simulink model "threebitsynupdowncounter"  (R2024a)
settings: Solver=VariableStepAuto  StartTime=0.0  StopTime=10.0  RelTol=1e-3
libraries: simulink_extras x4
settings Model: Creator=prath  LastModifiedBy=prath

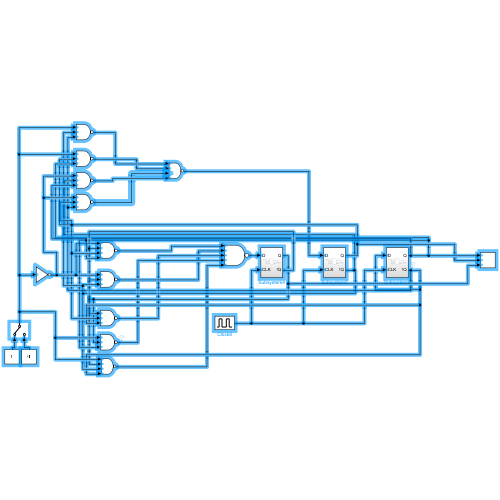
[thumbnail: Simulink's stored preview of the top-level diagram]
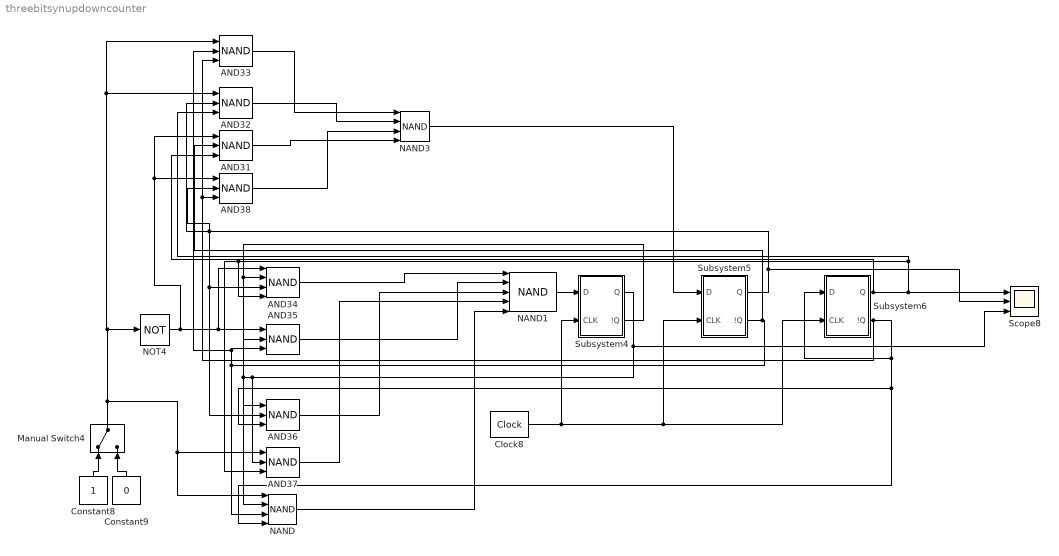
== system threebitsynupdowncounter ==
  AND{31..33,35..38} (7 alike) : Logic  Operator=NAND  Inputs=3  IconShape=distinctive  AllPortsSameDT=off  OutDataTypeStr=boolean
  AND34 : Logic  Operator=NAND  Inputs=4  IconShape=distinctive  AllPortsSameDT=off  OutDataTypeStr=boolean
  Clock8 : simulink_extras/Flip Flops/Clock  period=0.5
  Constant8 : Constant  OutDataTypeStr=boolean
  Constant9 : Constant  Value=0  OutDataTypeStr=boolean
  Manual Switch4 : ManualSwitch
  NAND : Logic  Operator=NAND  Inputs=4  IconShape=distinctive  AllPortsSameDT=off  OutDataTypeStr=boolean
  NAND1 : Logic  Operator=NAND  Inputs=5  IconShape=distinctive  AllPortsSameDT=off  OutDataTypeStr=boolean
  NAND3 : Logic  Operator=NAND  Inputs=4  IconShape=distinctive  AllPortsSameDT=off  OutDataTypeStr=boolean
  NOT4 : Logic  Operator=NOT  IconShape=distinctive  AllPortsSameDT=off  OutDataTypeStr=boolean
  Scope8 : Scope  NumInputPorts=3
  Subsystem4 : Subsystem
  Subsystem5 : Subsystem
  Subsystem6 : Subsystem
  wires:
  NAND/1 -> NAND1/5
  Clock8/1 -> Subsystem6/2(CLK), Subsystem5/2(CLK), Subsystem4/2(CLK)
  Subsystem5/2(!Q) -> AND31/2, AND35/3, AND33/2, NAND/3
  NOT4/1 -> AND38/1, AND31/1, AND35/1, AND34/1
  Subsystem5/1(Q) -> Scope8/2, AND32/2, AND36/2, AND34/3, AND38/2
  AND33/1 -> NAND3/1
  NAND3/1 -> Subsystem5/1(D)
  Subsystem6/2(!Q) -> AND38/3, AND33/3, AND36/3, NAND/4, Subsystem6/1(D)
  Manual Switch4/1 -> AND37/1, NAND/1, NOT4/1, AND32/1, AND33/1
  NAND1/1 -> Subsystem4/1(D)
  Subsystem6/1(Q) -> AND31/3, AND34/4, AND37/3, AND32/3, Scope8/1
  AND31/1 -> NAND3/4
  AND35/1 -> NAND1/2
  Constant9/1 -> Manual Switch4/2
  AND34/1 -> NAND1/1
  AND36/1 -> NAND1/3
  Subsystem4/1(Q) -> Scope8/3, AND37/2, AND36/1, AND35/2
  AND37/1 -> NAND1/4
  Subsystem4/2(!Q) -> NAND/2, AND34/2
  Constant8/1 -> Manual Switch4/1
  AND32/1 -> NAND3/2
  AND38/1 -> NAND3/3

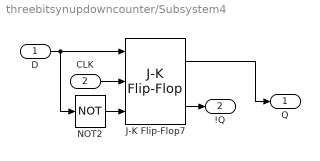
== system threebitsynupdowncounter/Subsystem4 ==
  D : Inport
  CLK : Inport  Port=2
  J-K Flip-Flop7 : simulink_extras/Flip Flops/J-K Flip-Flop  initial_condition=0
  NOT2 : Logic  Operator=NOT  IconShape=distinctive  AllPortsSameDT=off  OutDataTypeStr=boolean
  Q : Outport
  !Q : Outport  Port=2
  wires:
  NOT2/1 -> J-K Flip-Flop7/3
  J-K Flip-Flop7/2 -> !Q/1
  D/1 -> J-K Flip-Flop7/1, NOT2/1
  J-K Flip-Flop7/1 -> Q/1
  CLK/1 -> J-K Flip-Flop7/2

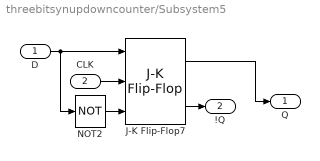
== system threebitsynupdowncounter/Subsystem5 ==
  D : Inport
  CLK : Inport  Port=2
  J-K Flip-Flop7 : simulink_extras/Flip Flops/J-K Flip-Flop  initial_condition=0
  NOT2 : Logic  Operator=NOT  IconShape=distinctive  AllPortsSameDT=off  OutDataTypeStr=boolean
  Q : Outport
  !Q : Outport  Port=2
  wires:
  NOT2/1 -> J-K Flip-Flop7/3
  J-K Flip-Flop7/2 -> !Q/1
  D/1 -> J-K Flip-Flop7/1, NOT2/1
  J-K Flip-Flop7/1 -> Q/1
  CLK/1 -> J-K Flip-Flop7/2

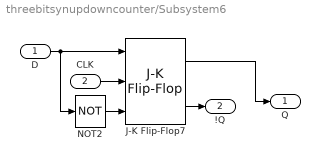
== system threebitsynupdowncounter/Subsystem6 ==
  D : Inport
  CLK : Inport  Port=2
  J-K Flip-Flop7 : simulink_extras/Flip Flops/J-K Flip-Flop  initial_condition=0
  NOT2 : Logic  Operator=NOT  IconShape=distinctive  AllPortsSameDT=off  OutDataTypeStr=boolean
  Q : Outport
  !Q : Outport  Port=2
  wires:
  NOT2/1 -> J-K Flip-Flop7/3
  J-K Flip-Flop7/2 -> !Q/1
  D/1 -> J-K Flip-Flop7/1, NOT2/1
  J-K Flip-Flop7/1 -> Q/1
  CLK/1 -> J-K Flip-Flop7/2
